simulink model "FrequencyDomain"  (R2022b)
settings: Solver=VariableStepAuto  StartTime=0.0  StopTime=600  RelTol=1e-3
values from neighbouring files (symbols this model uses):
  Dm = 7.59/1000    (= 0.00759)    [parameters.m]
  Dt = 15.8/100    (= 0.158)    [parameters.m]
  g = 9.81    [parameters.m]
  Jp = 2.15e-2    (= 0.0215)    [parameters.m]
  Jy = 2.37e-2    (= 0.0237)    [parameters.m]
  Mb = 1.075    [parameters.m]
undefined symbols (not defined in the file or in its folder): K_pitch, k_pitch, k_py, k_yaw, k_yp, w0_neg, w0_pos, w1_neg, w1_pos, w2_neg, w2_pos
libraries: cstblocks x2, SignalEditorBlockLib x2
settings Model: Creator=laptop  LastModifiedBy=lbend
settings SolverCC: AlgebraicLoopSolver=TrustRegion
settings OptimizationCC: BlockReduction=off  DefaultParameterBehavior=Inlined  BufferReuse=off
settings DebuggingCC: UnconnectedInputMsg=warning  UnconnectedOutputMsg=warning  UnconnectedLineMsg=warning  SFMachineParentedDataDiag=warning
settings ModelReferenceCC: EnableRefExpFcnMdlSchedulingChecks=on

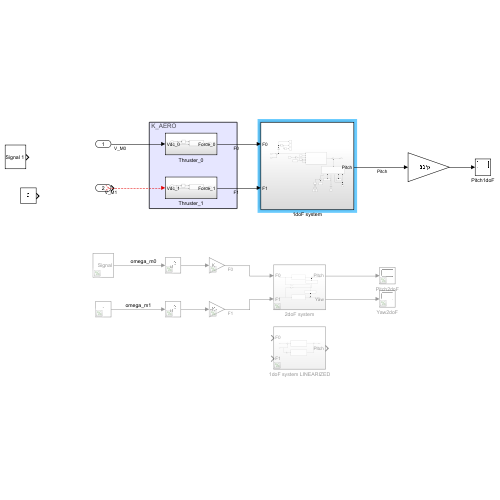
[thumbnail: Simulink's stored preview of the top-level diagram]
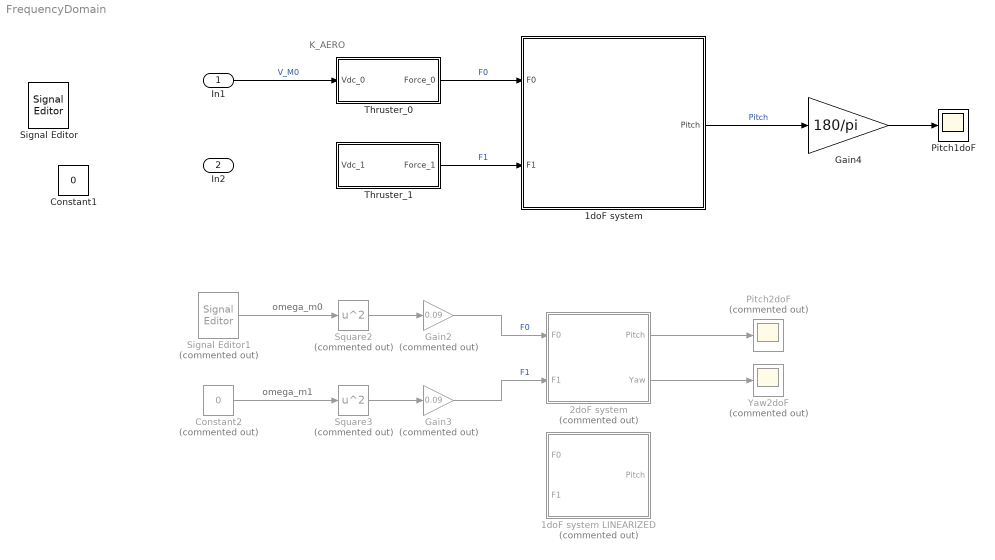
== system FrequencyDomain ==
  note: K_AERO
  note: omega_m1
  note: omega_m0
  In1 : Inport
  In2 : Inport  Port=2
  1doF system : Subsystem
  1doF system LINEARIZED : Subsystem  Commented=on
  2doF system : Subsystem  Commented=on
  Constant1 : Constant  Value=0
  Constant2 : Constant  Commented=on  Value=0
  Gain2 : Gain  Commented=on  Gain=0.09
  Gain3 : Gain  Commented=on  Gain=0.09
  Gain4 : Gain  Gain=180/pi
  Pitch1doF : Scope
  Pitch2doF : Scope  Commented=on
  Signal Editor : SignalEditorBlockLib/Signal Editor  FileName=C:\Users\laptop\Desktop\Automation and control laboratory\Helicopter\Helicopter\StepSignal30s.mat  ActiveScenario=Scenario  ActiveSignal=Signal  IsBus=off  OutputBusObjectStr=Bus: BusObject  SampleTime=0  Interpolate=off  ZeroCross=off  OutputAfterFinalValue=Setting to zero  Unit=inherit  PreserveSignalName=on
  Signal Editor1 : SignalEditorBlockLib/Signal Editor  Commented=on  FileName=C:\Users\lbend\OneDrive - Politecnico di Milano\Root Locos\MatLab&Simulink\StepSignal30s.mat  ActiveScenario=Scenario  ActiveSignal=Signal  IsBus=off  OutputBusObjectStr=Bus: BusObject  SampleTime=0  Interpolate=off  ZeroCross=off  OutputAfterFinalValue=Setting to zero  Unit=inherit  PreserveSignalName=on
  Square2 : Math  Commented=on  Operator=square
  Square3 : Math  Commented=on  Operator=square
  Thruster_0 : Subsystem
  Thruster_1 : Subsystem
  Yaw2doF : Scope  Commented=on
  wires:
  Thruster_0/1(Force_0) -> 1doF system/1(F0)  "F0"
  Thruster_1/1(Force_1) -> 1doF system/2(F1)  "F1"
  1doF system/1(Pitch) -> Gain4/1  "Pitch"
  2doF system/2(Yaw) -> Yaw2doF/1
  2doF system/1(Pitch) -> Pitch2doF/1
  Constant2/1 -> Square3/1
  Square3/1 -> Gain3/1
  Signal Editor1/1 -> Square2/1
  Square2/1 -> Gain2/1
  Gain2/1 -> 2doF system/1(F0)  "F0"
  Gain3/1 -> 2doF system/2(F1)  "F1"
  Gain4/1 -> Pitch1doF/1
  In1/1 -> Thruster_0/1(Vdc_0)  "V_M0"
  ? -> Thruster_1/1(Vdc_1)  "V_M1"

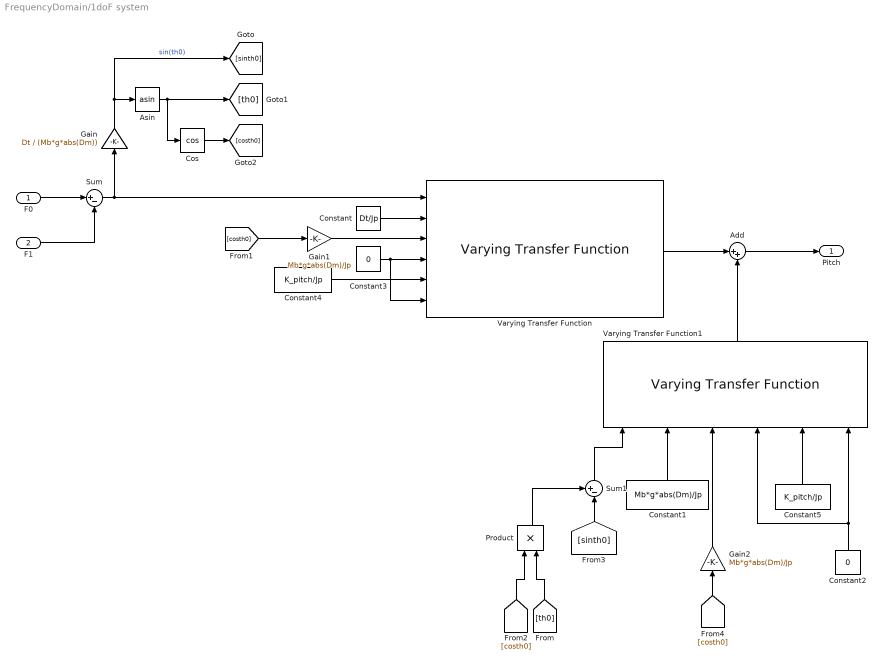
== system FrequencyDomain/1doF system ==
  F0 : Inport
  F1 : Inport  Port=2
  Add : Sum  Inputs=|++
  Asin : Trigonometry  Operator=asin
  Constant : Constant  Value=Dt/Jp
  Constant1 : Constant  Value=Mb*g*abs(Dm)/Jp
  Constant2 : Constant  Value=0
  Constant3 : Constant  Value=0
  Constant4 : Constant  Value=K_pitch/Jp
  Constant5 : Constant  Value=K_pitch/Jp
  Cos : Trigonometry  Operator=cos
  Gain : Gain  Gain=Dt / (Mb*g*abs(Dm))
  Gain1 : Gain  Gain=Mb*g*abs(Dm)/Jp
  Gain2 : Gain  Gain=Mb*g*abs(Dm)/Jp
  Product : Product
  Sum : Sum  Inputs=|+-
  Sum1 : Sum  Inputs=+-|
  Varying Transfer Function : cstblocks/Linear Parameter Varying/Varying Transfer Function  N=2
  Varying Transfer Function1 : cstblocks/Linear Parameter Varying/Varying Transfer Function  N=2
  Pitch : Outport
  wires:
  F0/1 -> Sum/1
  F1/1 -> Sum/2
  Add/1 -> Pitch/1
  Sum/1 -> Varying Transfer Function/1, Gain/1
  Gain/1 -> Asin/1, [sinth0]  "sin(th0)"
  Cos/1 -> [costh0]
  Gain2/1 -> Varying Transfer Function1/3
  Constant/1 -> Varying Transfer Function/2
  Constant1/1 -> Varying Transfer Function1/2
  Constant2/1 -> Varying Transfer Function1/6, Varying Transfer Function1/4
  Constant3/1 -> Varying Transfer Function/6, Varying Transfer Function/4
  Constant4/1 -> Varying Transfer Function/5
  Varying Transfer Function/1 -> Add/1
  Varying Transfer Function1/1 -> Add/2
  Sum1/1 -> Varying Transfer Function1/1
  Asin/1 -> [th0], Cos/1
  [sinth0] -> Sum1/2
  Product/1 -> Sum1/1
  [th0] -> Product/2
  [costh0] -> Product/1
  Constant5/1 -> Varying Transfer Function1/5
  [costh0] -> Gain1/1
  Gain1/1 -> Varying Transfer Function/3
  [costh0] -> Gain2/1

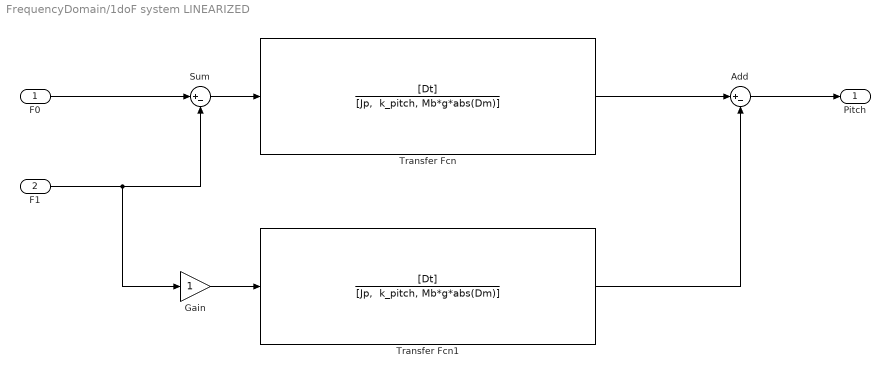
== system FrequencyDomain/1doF system LINEARIZED ==
  F0 : Inport
  F1 : Inport  Port=2
  Add : Sum  Inputs=|+-
  Gain : Gain
  Sum : Sum  Inputs=|+-
  Transfer Fcn : TransferFcn  Numerator=[Dt]  Denominator="[Jp,  k_pitch, Mb*g*abs(Dm)]"
  Transfer Fcn1 : TransferFcn  Numerator=[Dt]  Denominator="[Jp,  k_pitch, Mb*g*abs(Dm)]"
  Pitch : Outport
  wires:
  F0/1 -> Sum/1
  F1/1 -> Gain/1, Sum/2
  Sum/1 -> Transfer Fcn/1
  Transfer Fcn/1 -> Add/1
  Add/1 -> Pitch/1
  Transfer Fcn1/1 -> Add/2
  Gain/1 -> Transfer Fcn1/1

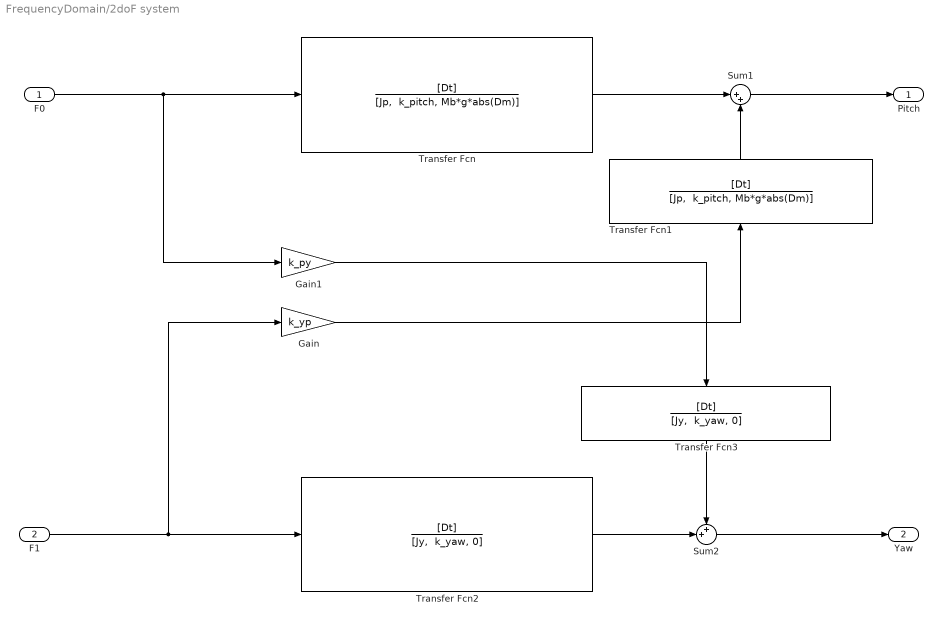
== system FrequencyDomain/2doF system ==
  F0 : Inport
  F1 : Inport  Port=2
  Gain : Gain  Gain=k_yp
  Gain1 : Gain  Gain=k_py
  Sum1 : Sum  Inputs=|++
  Sum2 : Sum  Inputs=++|
  Transfer Fcn : TransferFcn  Numerator=[Dt]  Denominator="[Jp,  k_pitch, Mb*g*abs(Dm)]"
  Transfer Fcn1 : TransferFcn  Numerator=[Dt]  Denominator="[Jp,  k_pitch, Mb*g*abs(Dm)]"
  Transfer Fcn2 : TransferFcn  Numerator=[Dt]  Denominator="[Jy,  k_yaw, 0]"
  Transfer Fcn3 : TransferFcn  Numerator=[Dt]  Denominator="[Jy,  k_yaw, 0]"
  Pitch : Outport
  Yaw : Outport  Port=2
  wires:
  F0/1 -> Gain1/1, Transfer Fcn/1
  Transfer Fcn/1 -> Sum1/1
  Transfer Fcn1/1 -> Sum1/2
  Sum1/1 -> Pitch/1
  F1/1 -> Gain/1, Transfer Fcn2/1
  Gain/1 -> Transfer Fcn1/1
  Gain1/1 -> Transfer Fcn3/1
  Sum2/1 -> Yaw/1
  Transfer Fcn2/1 -> Sum2/2
  Transfer Fcn3/1 -> Sum2/1

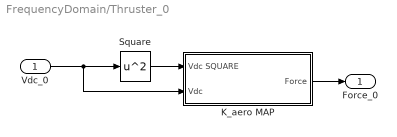
== system FrequencyDomain/Thruster_0 ==
  Vdc_0 : Inport
  K_aero MAP : Subsystem
  Square : Math  Operator=square
  Force_0 : Outport
  wires:
  Vdc_0/1 -> K_aero MAP/2(Vdc), Square/1
  Square/1 -> K_aero MAP/1(Vdc SQUARE)
  K_aero MAP/1(Force) -> Force_0/1

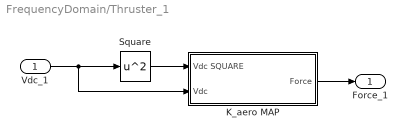
== system FrequencyDomain/Thruster_1 ==
  Vdc_1 : Inport
  K_aero MAP : Subsystem
  Square : Math  Operator=square
  Force_1 : Outport
  wires:
  Vdc_1/1 -> K_aero MAP/2(Vdc), Square/1
  Square/1 -> K_aero MAP/1(Vdc SQUARE)
  K_aero MAP/1(Force) -> Force_1/1

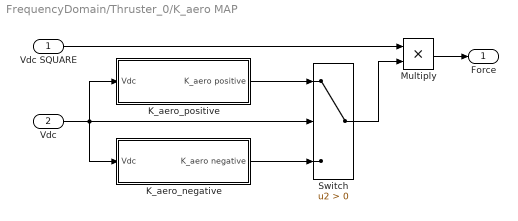
== system FrequencyDomain/Thruster_0/K_aero MAP ==
  Vdc SQUARE : Inport
  Vdc : Inport  Port=2
  K_aero_negative : Subsystem
  K_aero_positive : Subsystem
  "Multiply " : Product  Inputs=**
  Switch : Switch  Criteria=u2 > Threshold  SaturateOnIntegerOverflow=off  InputSameDT=off
  Force : Outport
  wires:
  Vdc SQUARE/1 -> "Multiply "/1
  "Multiply "/1 -> Force/1
  Vdc/1 -> K_aero_negative/1(Vdc), Switch/2, K_aero_positive/1(Vdc)
  K_aero_positive/1(K_aero positive) -> Switch/1
  K_aero_negative/1(K_aero negative) -> Switch/3
  Switch/1 -> "Multiply "/2

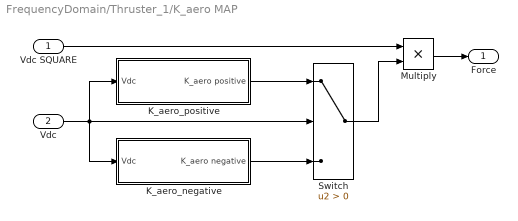
== system FrequencyDomain/Thruster_1/K_aero MAP ==
  Vdc SQUARE : Inport
  Vdc : Inport  Port=2
  K_aero_negative : Subsystem
  K_aero_positive : Subsystem
  "Multiply " : Product  Inputs=**
  Switch : Switch  Criteria=u2 > Threshold  SaturateOnIntegerOverflow=off  InputSameDT=off
  Force : Outport
  wires:
  Vdc SQUARE/1 -> "Multiply "/1
  "Multiply "/1 -> Force/1
  Vdc/1 -> K_aero_negative/1(Vdc), Switch/2, K_aero_positive/1(Vdc)
  K_aero_positive/1(K_aero positive) -> Switch/1
  K_aero_negative/1(K_aero negative) -> Switch/3
  Switch/1 -> "Multiply "/2

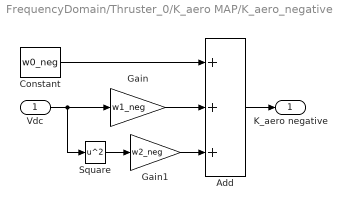
== system FrequencyDomain/Thruster_0/K_aero MAP/K_aero_negative ==
  Vdc : Inport
  Add : Sum  Inputs=+++
  Constant : Constant  Value=w0_neg
  Gain : Gain  Gain=w1_neg
  Gain1 : Gain  Gain=w2_neg
  Square : Math  Operator=square
  K_aero negative : Outport
  wires:
  Vdc/1 -> Square/1, Gain/1
  Gain1/1 -> Add/3
  Add/1 -> K_aero negative/1
  Constant/1 -> Add/1
  Gain/1 -> Add/2
  Square/1 -> Gain1/1

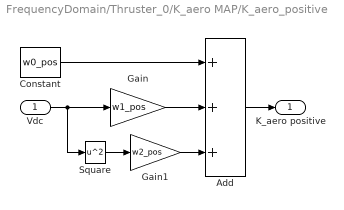
== system FrequencyDomain/Thruster_0/K_aero MAP/K_aero_positive ==
  Vdc : Inport
  Add : Sum  Inputs=+++
  Constant : Constant  Value=w0_pos
  Gain : Gain  Gain=w1_pos
  Gain1 : Gain  Gain=w2_pos
  Square : Math  Operator=square
  K_aero positive : Outport
  wires:
  Constant/1 -> Add/1
  Vdc/1 -> Square/1, Gain/1
  Add/1 -> K_aero positive/1
  Gain/1 -> Add/2
  Square/1 -> Gain1/1
  Gain1/1 -> Add/3

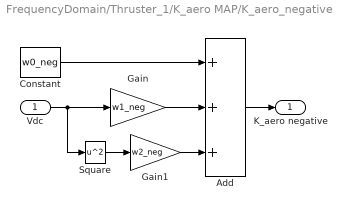
== system FrequencyDomain/Thruster_1/K_aero MAP/K_aero_negative ==
  Vdc : Inport
  Add : Sum  Inputs=+++
  Constant : Constant  Value=w0_neg
  Gain : Gain  Gain=w1_neg
  Gain1 : Gain  Gain=w2_neg
  Square : Math  Operator=square
  K_aero negative : Outport
  wires:
  Vdc/1 -> Square/1, Gain/1
  Gain1/1 -> Add/3
  Add/1 -> K_aero negative/1
  Constant/1 -> Add/1
  Gain/1 -> Add/2
  Square/1 -> Gain1/1

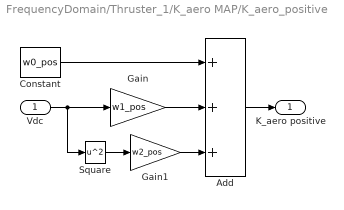
== system FrequencyDomain/Thruster_1/K_aero MAP/K_aero_positive ==
  Vdc : Inport
  Add : Sum  Inputs=+++
  Constant : Constant  Value=w0_pos
  Gain : Gain  Gain=w1_pos
  Gain1 : Gain  Gain=w2_pos
  Square : Math  Operator=square
  K_aero positive : Outport
  wires:
  Constant/1 -> Add/1
  Vdc/1 -> Square/1, Gain/1
  Add/1 -> K_aero positive/1
  Gain/1 -> Add/2
  Square/1 -> Gain1/1
  Gain1/1 -> Add/3
